simulink model "fase2_lazo_cerrado"  (R2021a)
settings: Solver=ode45  StartTime=0.0  StopTime=5  RelTol=1e-3
values from neighbouring files (symbols this model uses):
  A = double(subs(A_lin, p_syms, p_vals))    [fase1_modelado.m]    (also in fase4_barrido_rodilla.m = [0 1 0 0; 0 0 -bet*Mb*g*L/dt_ 0; 0 0 0 1; 0 0 alp*Mb*g*L/dt_; lqr_design.mat = [0 0 0 0 1 0 0 0 0 -8.61714614499 0 78.7721246338 ... (16 el; modelo_robot.mat = [0 0 0 0 1 0 0 0 0 -8.61714614499 0 78.7721246338 ... (16 el)
  B = double(subs(B_lin, p_syms, p_vals))    [fase1_modelado.m]    (also in fase4_barrido_rodilla.m = [0; (J/R+bet)/dt_; 0; -(alp+bet/R)/dt_]; lqr_design.mat = [0 27.4685928751 0 -140.962873143]; modelo_robot.mat = [0 27.4685928751 0 -140.962873143])
  C = eye(4)    [fase1_modelado.m]    (also in fase3_analiza_catch.m = C(all(~isnan(C),2), :); lqr_design.mat = [1 0 0 0 0 1 0 0 0 0 1 0 ... (16 elements, 4x4)]; modelo_robot.mat = [1 0 0 0 0 1 0 0 0 0 1 0 ... (16 elements, 4x4)])
  D = zeros(4,1)    [fase1_modelado.m]    (also in fase3_plot_ocho.m = D(all(~isnan(D),2), :); fase3_zoom_fin.m = D(all(~isnan(D),2), :); lqr_design.mat = [0 0 0 0]; modelo_robot.mat = [0 0 0 0])
  Kd = dlqr(Ad, Bd, Qlqr, Rlqr)    [fase2_lqr.m]    (also in lqr_design.mat = [-0.681886355 -1.22830555376 -6.85943769697 -0.816592230514])
  Ts = 0.01    [fase2_lqr.m]    (also in lqr_design.mat)
settings Model: Creator=luisf  LastModifiedBy=luisf

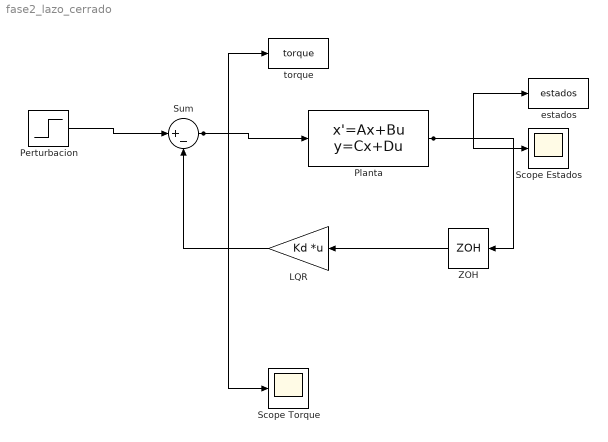
== system fase2_lazo_cerrado ==
  LQR : Gain  Gain=Kd  Multiplication=Matrix(K*u)
  Perturbacion : Step  After=0.3  SampleTime=0
  Planta : StateSpace  A=A  B=B  C=C  D=D  InitialCondition=[0; 0; 0.05; 0]
  Scope Estados : Scope
  Scope Torque : Scope
  Sum : Sum  Inputs=|+-
  ZOH : ZeroOrderHold  SampleTime=Ts
  estados : ToWorkspace  VariableName=estados  SaveFormat=Timeseries  SampleTime=-1
  torque : ToWorkspace  VariableName=torque  SaveFormat=Timeseries  SampleTime=-1
  wires:
  Perturbacion/1 -> Sum/1
  Sum/1 -> Planta/1, torque/1, Scope Torque/1
  Planta/1 -> ZOH/1, estados/1, Scope Estados/1
  ZOH/1 -> LQR/1
  LQR/1 -> Sum/2
